simulink model "untitled"  (R2019a)
settings: Solver=VariableStepAuto  StartTime=0.0  StopTime=22.46  RelTol=1e-3
values from neighbouring files (symbols this model uses):
  B = b*dt    [Kalman_test.m]    (also in MRAC.m = [0 ;w0^2]; MRAC2.m = [0 ;w0^2]; Untitled5.m = [0 w0^2])
settings Model: Creator=Student  LastModifiedBy=Student

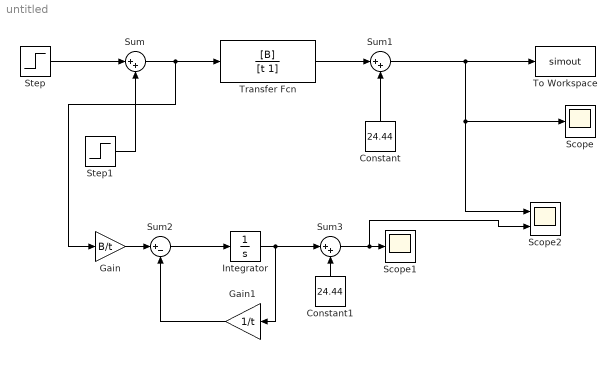
== system untitled ==
  Constant : Constant  Value=24.44
  Constant1 : Constant  Value=24.44
  Gain : Gain  Gain=B/t
  Gain1 : Gain  Gain=1/t
  Integrator : Integrator
  Scope : Scope
  Scope1 : Scope
  Scope2 : Scope  NumInputPorts=2
  Step : Step  After=-1.075  SampleTime=0
  Step1 : Step  Time=11  After=1.075  SampleTime=0
  Sum : Sum  Inputs=|++
  Sum1 : Sum  Inputs=|++
  Sum2 : Sum  Inputs=|+-
  Sum3 : Sum  Inputs=|++
  To Workspace : ToWorkspace  VariableName=simout  SaveFormat=Timeseries  SampleTime=-1
  Transfer Fcn : TransferFcn  Numerator=[B]  Denominator=[t 1]
  wires:
  Step/1 -> Sum/1
  Sum/1 -> Gain/1, Transfer Fcn/1
  Step1/1 -> Sum/2
  Transfer Fcn/1 -> Sum1/1
  Constant/1 -> Sum1/2
  Sum1/1 -> To Workspace/1, Scope2/1, Scope/1
  Integrator/1 -> Sum3/1, Gain1/1
  Gain1/1 -> Sum2/2
  Gain/1 -> Sum2/1
  Sum2/1 -> Integrator/1
  Sum3/1 -> Scope2/2, Scope1/1
  Constant1/1 -> Sum3/2
